simulink model "MPC_Sim"  (R2020a)
settings: Solver=FixedStepAuto  StartTime=0.0  StopTime=100  FixedStep=1e-2  RelTol=1e-3
settings Model: Creator=niran  LastModifiedBy=niranjan.bhujel

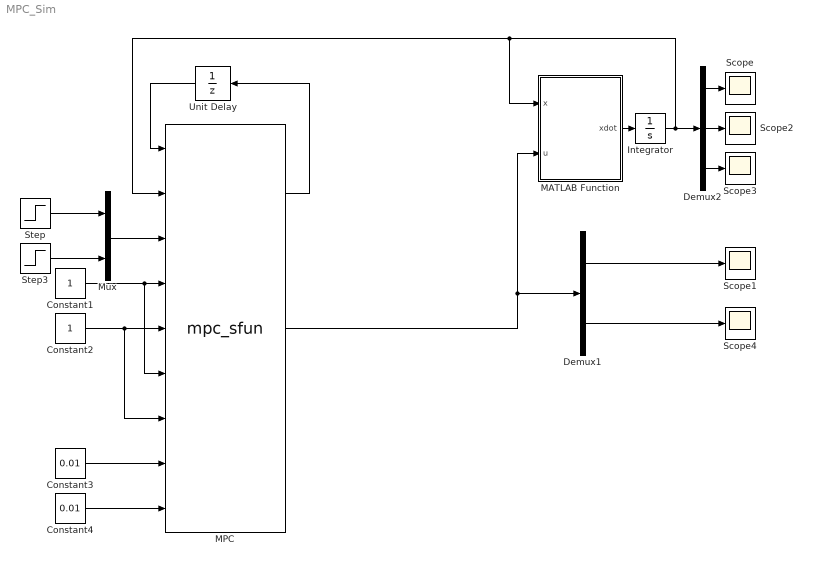
== system MPC_Sim ==
  Constant1 : Constant
  Constant2 : Constant
  Constant3 : Constant  Value=0.01
  Constant4 : Constant  Value=0.01
  Demux1 : Demux  Outputs=2
  Demux2 : Demux  Outputs=3
  Integrator : Integrator
  MATLAB Function : MATLAB Function  TreatAsAtomicUnit=on
  MPC : S-Function  InitFcn=try, set_param(gcb,'FunctionName','mpc_sfun'), end  FunctionName=mpc_sfun  SFunctionModules=mpc_sfun_wrapper MPC_Code MPC_Code_Call  SFunctionDeploymentMode=off  EnableBusSupport=off  mask(S-Function Builder){}
      mask help: Simulink:masks:SFunctionBuilder_MD
      mask init:
      | val = [[.9  0.75 0.75 1 1 .9 .9 1]',[1 1 0.75 0.75 .9 .9 1 .9]'];try , sys = get_param(gcb,'SfunBuilderFcnName');if isempty(sys), sys = get_param(gcb,'FunctionName'); end,catch, sys = get_param(gcb,'FunctionName'); end
      settings: CopyFcn=set_param(gcbh,'LinkStatus','none')  PreSaveFcn=try, set_param(gcb,'FunctionName','mpc_sfun'), end  OpenFcn=sfunctionwizard(gcbh)
      mask Display: plot(val(:,1),val(:,2)),disp(sys), port_label('input',1,'zGuess'), port_label('input',2,'x0'), port_label('input',3,'xref'), port_label('input',4,'Qp11'), port_label('input',5,'Qp22'), port_label('input',6,'Qtp11'), port_label('input',7,'Qtp22'), port_label('input',8,'Rp11'), port_label('input',9,'Rp22'), port_label('output',1,'zOut'), port_label('output',2,'uCalc'), port_label('output',3,'Cost')
  Mux : Mux  Inputs=2
  Scope{,1..4} (5 alike) : Scope
  Step : Step  Time=50  Before=0.5  SampleTime=0
  Step3 : Step  Time=75  Before=25  After=35  SampleTime=0
  Unit Delay : UnitDelay  SampleTime=-1  HasFrameUpgradeWarning=on
  wires:
  MPC/2 -> MATLAB Function/2(u), Demux1/1
  Demux1/1 -> Scope1/1
  Demux1/2 -> Scope4/1
  MATLAB Function/1(xdot) -> Integrator/1
  Demux2/1 -> Scope/1
  Demux2/2 -> Scope2/1
  Demux2/3 -> Scope3/1
  MPC/1 -> Unit Delay/1
  Unit Delay/1 -> MPC/1
  Constant1/1 -> MPC/6, MPC/4
  Constant2/1 -> MPC/7, MPC/5
  Constant3/1 -> MPC/8
  Step/1 -> Mux/1
  Step3/1 -> Mux/2
  Mux/1 -> MPC/3
  Constant4/1 -> MPC/9
  Integrator/1 -> MATLAB Function/1(x), MPC/2, Demux2/1

== matlab function MPC_Sim/MATLAB Function ==
  data: x input; u input; xdot output
function xdot = fcn(x, u)
    xdot = zeros(3, 1);
    A = [-0.4, 0.1, -2.0;
        0, -0.3, 4.0;
        1.0, 0.0, 0.0];
    B = [1, 1;
        0, 1;
        1, 0];
    
    xdot = A * x + B * u;
end
